simulink model "sim_project"  (R2021a)
settings: Solver=VariableStepAuto  StartTime=0.0  StopTime=10.0  RelTol=1e-3
settings Model: Creator=Abd-Elrahman Zidan  LastModifiedBy=Abd-Elrahman Zidan

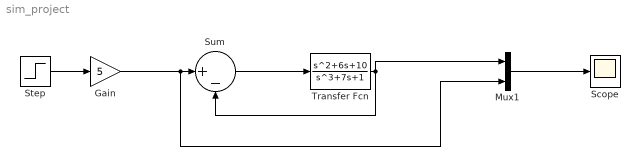
== system sim_project ==
  Gain : Gain  Gain=5
  Mux1 : Mux  Inputs=2
  Scope : Scope
  Step : Step  SampleTime=0
  Sum : Sum  Inputs=|+-
  Transfer Fcn : TransferFcn  Numerator=[1 6 10]  Denominator=[1 0 7 1]
  wires:
  Sum/1 -> Transfer Fcn/1
  Mux1/1 -> Scope/1
  Step/1 -> Gain/1
  Transfer Fcn/1 -> Sum/2, Mux1/1
  Gain/1 -> Mux1/2, Sum/1
